simulink model "Ex3_2_4"  (R2022b)
settings: Solver=VariableStepAuto  StartTime=0.0  StopTime=25  RelTol=1e-3
settings Model: Creator=15043  LastModifiedBy=15043

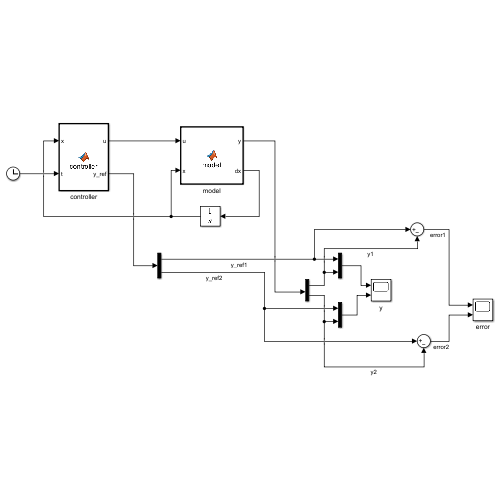
[thumbnail: Simulink's stored preview of the top-level diagram]
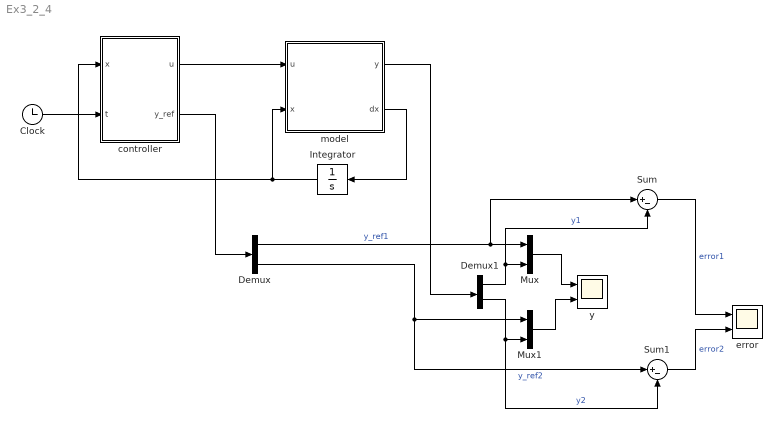
== system Ex3_2_4 ==
  Clock : Clock
  Demux : Demux  Outputs=2
  Demux1 : Demux  Outputs=2
  Integrator : Integrator  InitialCondition=[0;0;0;0;0;]
  Mux : Mux  Inputs=2
  Mux1 : Mux  Inputs=2
  Sum : Sum  Inputs=|+-
  Sum1 : Sum  Inputs=|+-
  controller : MATLAB Function  TreatAsAtomicUnit=on
  error : Scope  NumInputPorts=2
  model : MATLAB Function  TreatAsAtomicUnit=on
  y : Scope  NumInputPorts=2
  wires:
  controller/1(u) -> model/1(u)
  Clock/1 -> controller/2(t)
  model/2(dx) -> Integrator/1
  Integrator/1 -> model/2(x), controller/1(x)
  Demux/2 -> Mux1/1, Sum1/1  "y_ref2"
  Sum/1 -> error/1  "error1"
  Sum1/1 -> error/2  "error2"
  Demux/1 -> Mux/1, Sum/1  "y_ref1"
  Mux1/1 -> y/2
  Demux1/2 -> Mux1/2, Sum1/2  "y2"
  Demux1/1 -> Mux/2, Sum/2  "y1"
  Mux/1 -> y/1
  controller/2(y_ref) -> Demux/1
  model/1(y) -> Demux1/1

== matlab function Ex3_2_4/controller ==
  data: x input; u output; t input; y_ref output
function [u,y_ref] = controller(x,t)
%#codegen

%    This function was generated by the Symbolic Math Toolbox version 9.2.
%    30-Nov-2022 21:05:51

x1 = x(1,:);
x2 = x(2,:);
x3 = x(3,:);
x4 = x(4,:);
u = [t.*(3.0./2.5e+1)+x1-x3.*2.0+t.^2.*(6.0./1.25e+2)-t.^3./2.5e+2;t.*(9.0./5.0e+1)-x2-x4-x1.*x3+t.^2.*(9.0./1.25e+2)-t.^3.*(3.0./5.0e+2)];
if nargout > 1
    y_ref = [t.^2.*(3.0./5.0e+1)-t.^3./2.5e+2;t.^2.*(9.0./1.0e+2)-t.^3.*(3.0./5.0e+2)];
end

== matlab function Ex3_2_4/model ==
  data: u input; y output; x input; dx output
function [y,dx] = model(u,x)
%#codegen

%    This function was generated by the Symbolic Math Toolbox version 9.2.
%    30-Nov-2022 21:05:52

u1 = u(1,:);
u2 = u(2,:);
x1 = x(1,:);
x2 = x(2,:);
x3 = x(3,:);
x4 = x(4,:);
x5 = x(5,:);
y = [x3;x2];
if nargout > 1
    dx = [-x1+x2.^2;u2+x4+x1.*x3;u1-x1+x3;u1+x5;-x5+u1.*x2+x3.^2];
end
